simulink model "test12"  (R2022a)
settings: Solver=VariableStepAuto  StartTime=0.0  StopTime=10.0  RelTol=1e-3
settings Model: Creator=ygkwon  LastModifiedBy=ygkwon

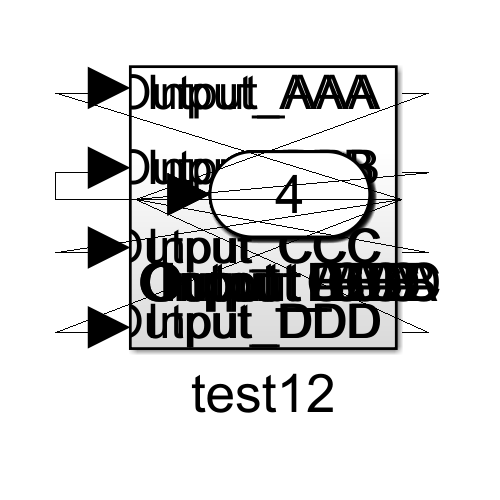
[thumbnail: Simulink's stored preview of the top-level diagram]
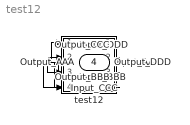
== system test12 ==
  Input_AAA : Inport
  Input_BBB : Inport  Port=2
  Input_CCC : Inport  Port=3
  Input_DDD : Inport  Port=4
  test12 : Subsystem
  Output_AAA : Outport
  Output_BBB : Outport  Port=2
  Output_CCC : Outport  Port=3
  Output_DDD : Outport  Port=4
  wires:
  Input_AAA/1 -> test12/1(Input_AAA)
  Input_BBB/1 -> test12/2(Input_BBB)
  Input_CCC/1 -> test12/3(Input_CCC)
  Input_DDD/1 -> test12/4(Input_DDD)
  test12/1(Output_AAA) -> Output_AAA/1
  test12/2(Output_BBB) -> Output_BBB/1
  test12/3(Output_CCC) -> Output_CCC/1
  test12/4(Output_DDD) -> Output_DDD/1

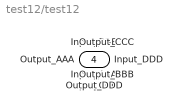
== system test12/test12 ==
  Input_AAA : Inport
  Input_BBB : Inport  Port=2
  Input_CCC : Inport  Port=3
  Input_DDD : Inport  Port=4
  Output_AAA : Outport
  Output_BBB : Outport  Port=2
  Output_CCC : Outport  Port=3
  Output_DDD : Outport  Port=4
